simulink model "RRRTask1Dynamics"  (R2018b)
settings: Solver=VariableStepAuto  StartTime=0.0  StopTime=inf  RelTol=1e-3
settings Model: Creator=Young Wang  LastModifiedBy=Young Wang

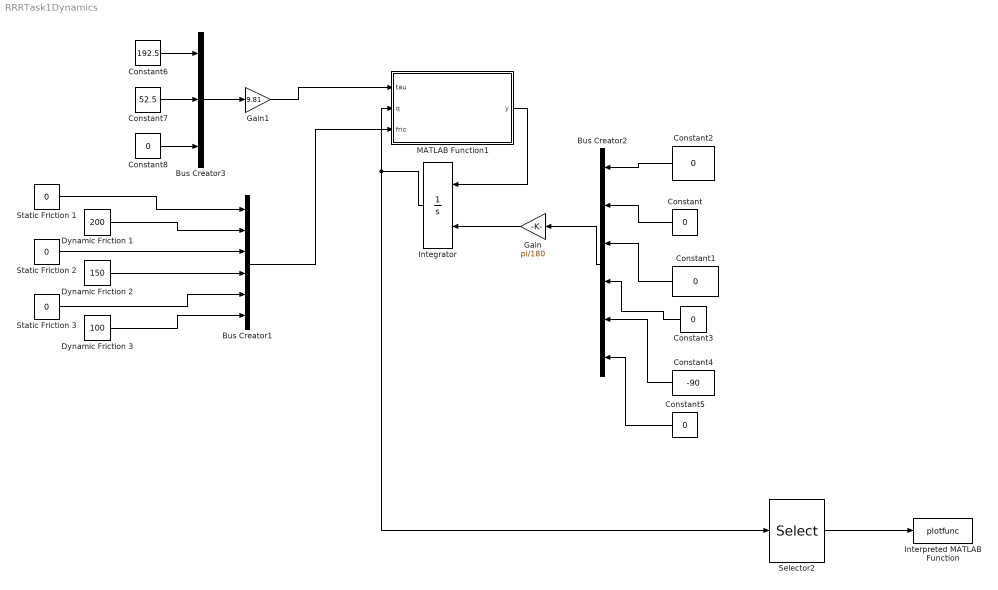
== system RRRTask1Dynamics ==
  Bus Creator1 : BusCreator  Inputs=6
  Bus Creator3 : BusCreator  Inputs=3
  Bus Creator2 : BusCreator  Inputs=6
  Constant{,1..3,5,8} (6 alike) : Constant  Value=0
  Constant4 : Constant  Value=-90
  Constant6 : Constant  Value=192.5
  Constant7 : Constant  Value=52.5
  Dynamic Friction 1 : Constant  Value=200
  Dynamic Friction 2 : Constant  Value=150
  Dynamic Friction 3 : Constant  Value=100
  Gain : Gain  Gain=pi/180
  Gain1 : Gain  Gain=9.81
  Integrator : Integrator  InitialConditionSource=external
  Interpreted MATLAB Function : MATLABFcn  MATLABFcn=plotfunc  OutputDimensions=0
  MATLAB Function1 : MATLAB Function  TreatAsAtomicUnit=on
  Selector2 : Selector  InputPortWidth=6  IndexOptions=Index vector (dialog)  Indices=[1 3 5]  OutputSizes=1
  Static Friction 1 : Constant  Value=0
  Static Friction 2 : Constant  Value=0
  Static Friction 3 : Constant  Value=0
  wires:
  MATLAB Function1/1(y) -> Integrator/1
  Constant4/1 -> Bus Creator2/5
  Constant5/1 -> Bus Creator2/6
  Constant1/1 -> Bus Creator2/3
  Bus Creator2/1 -> Gain/1
  Constant2/1 -> Bus Creator2/1
  Selector2/1 -> Interpreted MATLAB Function/1
  Constant/1 -> Bus Creator2/2
  Constant3/1 -> Bus Creator2/4
  Integrator/1 -> Selector2/1, MATLAB Function1/2(q)
  Dynamic Friction 1/1 -> Bus Creator1/2
  Dynamic Friction 2/1 -> Bus Creator1/4
  Static Friction 1/1 -> Bus Creator1/1
  Static Friction 2/1 -> Bus Creator1/3
  Dynamic Friction 3/1 -> Bus Creator1/6
  Static Friction 3/1 -> Bus Creator1/5
  Bus Creator1/1 -> MATLAB Function1/3(fric)
  Constant6/1 -> Bus Creator3/1
  Constant7/1 -> Bus Creator3/2
  Constant8/1 -> Bus Creator3/3
  Bus Creator3/1 -> Gain1/1
  Gain/1 -> Integrator/2
  Gain1/1 -> MATLAB Function1/1(tau)

== matlab function RRRTask1Dynamics/MATLAB Function1 ==
  data: tau input; y output; q input; fric input
function y = Dynamics(tau,q,fric)
%parsing q
q1=q(1);
q1dot=q(2);
q2=q(3);
q2dot=q(4);
q3=q(5);
q3dot=q(6);

%Friction Static and Dynamic
SF1 = fric(1);
SF2 = fric(3);
SF3 = fric(5);
DF1 = fric(2);
DF2 = fric(4);
DF3 = fric(6);
%Mass matrix
M = zeros(3);
M(1,1) = 80*cos(q2+q3) + 420*cos(q2) + 60*cos(q3) + (12291/20);
M(1,2) = 40*cos(q2+q3) + 210*cos(q2) + 60*cos(q3) + (2681/20);
M(1,3) = 40*cos(q2+q3) + 30*cos(q3) + (101/10);
M(2,1) = 40*cos(q2+q3) + 210*cos(q2) + 60*cos(q3) + (2681/20);
M(2,2) = 60*cos(q3) + (2681/20);
M(2,3) = 30*cos(q3) + (101/10);
M(3,1) = 40*cos(q2+q3) + 30*cos(q3) + (101/10);
M(3,2) = 30*cos(q3) + (101/10);
M(3,3) = 101/10;

%C matrix
C = zeros(3);
C(1,2) = -40*sin(q2+q3) - 210*sin(q2);
C(1,3) = -40*sin(q2+q3) - 30*sin(q3);
C(2,1) = 40*sin(q2+q3) + 210*sin(q2);
C(2,3) = -30*sin(q3);
C(3,1) = 40*cos(q2+q3) + 30*sin(q3);
C(3,2) = 30*sin(q3);

%B matrix
B = zeros(3);
B(1,1) = -80*sin(q2+q3) - 420*sin(q2);
B(1,2) = -80*sin(q2+q3) -60*sin(q3);
B(1,3) = -80*sin(q2+q3) -60*sin(q3);
B(2,2) = -60*sin(q3);
B(2,3) = -60*sin(q3);
B(3,1) = 60*sin(q3);

%G matrix
g = 9.81;
G = [0;0;0];
G(1) = (5*g*(4*cos(q1 + q2 + q3) + 21*cos(q1 + q2) + 56*cos(q1)))/2;
G(2) = (105*g*cos(q1 + q2))/2 + 10*g*cos(q1 + q2 + q3);
G(3) = 10*g*cos(q1 + q2 + q3);

%F matrix
F = [0;0;0];
F(1)=SF1*sign(q1dot)+DF1*q1dot;
F(2)=SF2*sign(q2dot)+DF2*q2dot;
F(3)=SF3*sign(q3dot)+DF3*q3dot;

%Solving for acceleration
V=C*[q1dot;q2dot;q3dot].^2+B*[q1dot*q2dot;q1dot*q3dot;q2dot*q3dot];
qdd=pinv(M)*(tau-V-G-F);
y=[q1dot;qdd(1);q2dot;qdd(2);q3dot;qdd(3)];
end
